simulink model "Semi_Lead_Guidance_Method_6"  (R2024b)
settings: Solver=FixedStepAuto  StartTime=0.0  StopTime=200  FixedStep=0.01  RelTol=1e-3
values from neighbouring files (symbols this model uses):
  P = 2    [AAZ.m]    (also in TP3_1_6.m = P_values(idx))
settings Model: Creator=Acer  LastModifiedBy=Acer
settings DataIOCC: ReturnWorkspaceOutputs=off

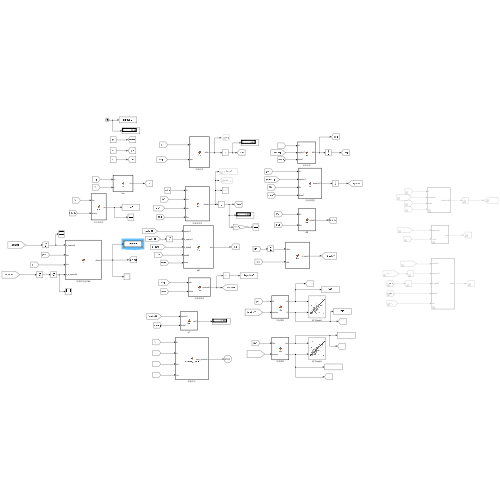
[thumbnail: Simulink's stored preview of the top-level diagram]
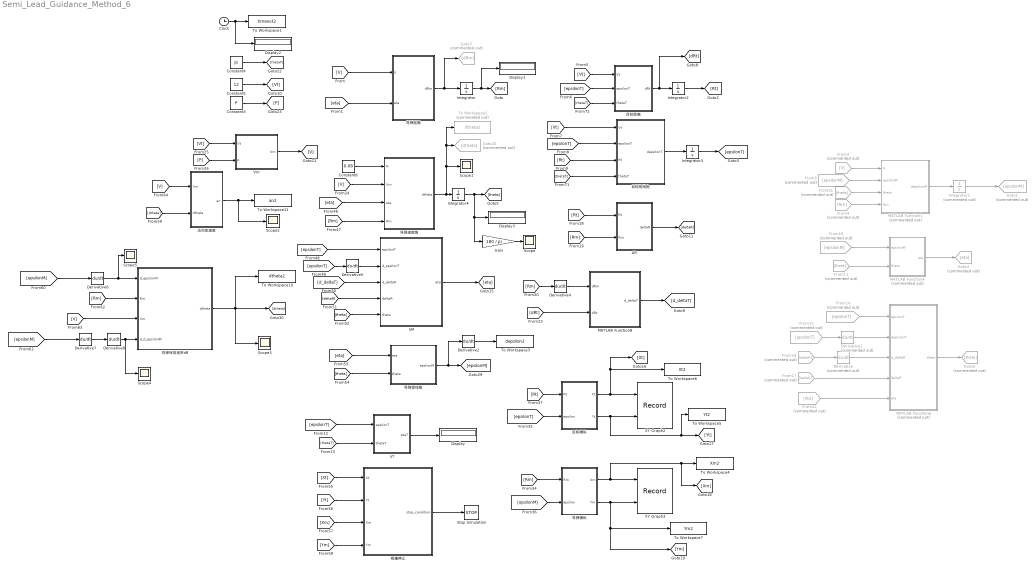
== system Semi_Lead_Guidance_Method_6 ==
  Clock : Clock
  Constant3 : Constant  Value=P
  Constant4 : Constant  Value=pi
  Constant5 : Constant  Value=12
  Constant6 : Constant  Value=0.08
  Derivative : Derivative  Commented=on
  Derivative1 : Derivative  Commented=on
  Derivative{2,4..8} (6 alike) : Derivative
  Display{,1..3} (4 alike) : Display
  From10 : From  Commented=on  GotoTag=epsilonM
  From11 : From  Commented=on  GotoTag=theta
  From14 : From  Commented=on  GotoTag=epsilonT
  From15 : From  Commented=on  GotoTag=epsilonT
  From16 : From  Commented=on  GotoTag=deltaR
  From17 : From  Commented=on  GotoTag=deltaR
  From2 : From  Commented=on  GotoTag=V
  From21 : From  Commented=on  GotoTag=theta
  From22 : From  Commented=on  GotoTag=eta
  From3 : From  Commented=on  GotoTag=epsilonM
  From4 : From  Commented=on  GotoTag=Rm
  Gain : Gain  Gain=180 / pi
  Goto1 : Goto  Commented=on  GotoTag=epsilonM
  Goto20 : Goto  Commented=on  GotoTag=dtheta
  Goto4 : Goto  Commented=on  GotoTag=eta
  Goto6 : Goto  Commented=on  GotoTag=theta
  Goto7 : Goto  Commented=on  GotoTag=dRm
  Integrator : Integrator  InitialCondition=50
  Integrator1 : Integrator  Commented=on  InitialCondition=65*pi/180
  Integrator2 : Integrator  InitialCondition=3000
  Integrator3 : Integrator  InitialCondition=70 * pi / 180
  Integrator4 : Integrator  InitialCondition=70 * pi /180
  MATLAB Function1 : MATLAB Function  Commented=on  TreatAsAtomicUnit=on
  MATLAB Function4 : MATLAB Function  Commented=on  TreatAsAtomicUnit=on
  MATLAB Function6 : MATLAB Function  Commented=on  TreatAsAtomicUnit=on
  MATLAB Function8 : MATLAB Function  TreatAsAtomicUnit=on
  Scope{,1..5} (6 alike) : Scope
  Stop Simulation : Stop
  To Workspace1 : ToWorkspace  VariableName=timeout2  SaveFormat=Timeseries  SampleTime=-1
  To Workspace10 : ToWorkspace  VariableName=dtheta2  SaveFormat=Timeseries  SampleTime=-1
  To Workspace11 : ToWorkspace  VariableName=an2  SaveFormat=Timeseries  SampleTime=-1
  To Workspace2 : ToWorkspace  Commented=on  VariableName=dtheta2  SaveFormat=Timeseries  SampleTime=-1
  To Workspace3 : ToWorkspace  VariableName=depsilon2  SaveFormat=Timeseries  SampleTime=-1
  To Workspace4 : ToWorkspace  VariableName=Xm2  SaveFormat=Timeseries  SampleTime=-1
  To Workspace5 : ToWorkspace  VariableName=Yt2  SaveFormat=Timeseries  SampleTime=-1
  To Workspace6 : ToWorkspace  VariableName=Xt2  SaveFormat=Timeseries  SampleTime=-1
  To Workspace7 : ToWorkspace  VariableName=Ym2  SaveFormat=Timeseries  SampleTime=-1
  Vm : MATLAB Function  TreatAsAtomicUnit=on
  XY Graph2 : Record  FileSettingsInternal="{\"entries\":[{\"content\":{\"excelSettings\":{\"content\":{},\"type\":\"Streamout.ExcelSettings\"}},\"type\":\"Streamout.FileSettingStorage\",\"uuid\":\"\"}],\"packageUris\":[\"http:\\/\\/schema.mathworks.com\\/mf0\\/streamout_blocks\\/R2020a\"],\"version\":\"1.0\"}"  Layout=[1 1]  SignalsInternal="{\"entries\":[{\"content\":{\"signals\":[{\"content\":{\"blockPath\":[],\"dimensions\":[1],\"domain\":\"\",\"lineColor\":\"#b746ff\",\"lineWidth\":2,\"plots\":[ 1 ],\"port\":1,\"sid\":[\"\"],\"signalID\":1,\"signalName\":\"目标横纵:1\"},\"type\":\"RecordBlkView.Signal\",\"uuid\":\"\"},{\"content\":{\"blockPath\":[],\"dimensions\":[1],\"domain\":\"\",\"lineColor\":\"#64d413\",\"lineWidth\":2,\"plots\":[ 1 ],\"port\":2,\"sid\":[\"\"],\"signalID\":2,\"signalName\":\"目标横纵:2\"},\"type\":\"RecordBlkView.Signal\",\"uuid\":\"\"}]},\"type\":\"RecordBlkView.InputSignals\",\"uuid\":\"\"}],\"packageUris\":[\"http:\\/\\/schema.mathworks.com\\/mf0\\/streamout_blocks\\/R2020a\"],\"version\":\"1.0\"}"  VisualizationBindings="{\"xyplotplugin\":{\"info\":[{\"series\":[{\"bindingParametersList\":[{\"parameter\":\"X-Axis\",\"signalID\":1,\"signalName\":\"目标横纵:1\"},{\"parameter\":\"Y-Axis\",\"signalID\":2,\"signalName\":\"目标横纵:2\"}],\"seriesID\":0}],\"subplotID\":1}]}}"  CompatibilityTag=XY
  XY Graph3 : Record  FileSettingsInternal="{\"entries\":[{\"content\":{\"excelSettings\":{\"content\":{},\"type\":\"Streamout.ExcelSettings\"}},\"type\":\"Streamout.FileSettingStorage\",\"uuid\":\"\"}],\"packageUris\":[\"http:\\/\\/schema.mathworks.com\\/mf0\\/streamout_blocks\\/R2020a\"],\"version\":\"1.0\"}"  Layout=[1 1]  SignalsInternal="{\"entries\":[{\"content\":{\"signals\":[{\"content\":{\"blockPath\":[],\"dimensions\":[1],\"domain\":\"\",\"lineColor\":\"#ff13a6\",\"lineWidth\":2,\"plots\":[ 1 ],\"port\":1,\"sid\":[\"\"],\"signalID\":1,\"signalName\":\"导弹横纵:1\"},\"type\":\"RecordBlkView.Signal\",\"uuid\":\"\"},{\"content\":{\"blockPath\":[],\"dimensions\":[1],\"domain\":\"\",\"lineColor\":\"#fe330a\",\"lineWidth\":2,\"plots\":[ 1 ],\"port\":2,\"sid\":[\"\"],\"signalID\":2,\"signalName\":\"导弹横纵:2\"},\"type\":\"RecordBlkView.Signal\",\"uuid\":\"\"}]},\"type\":\"RecordBlkView.InputSignals\",\"uuid\":\"\"}],\"packageUris\":[\"http:\\/\\/schema.mathworks.com\\/mf0\\/streamout_blocks\\/R2020a\"],\"version\":\"1.0\"}"  VisualizationBindings="{\"xyplotplugin\":{\"info\":[{\"series\":[{\"bindingParametersList\":[{\"parameter\":\"X-Axis\",\"signalID\":1,\"signalName\":\"导弹横纵:1\"},{\"parameter\":\"Y-Axis\",\"signalID\":2,\"signalName\":\"导弹横纵:2\"}],\"seriesID\":0}],\"subplotID\":1}]}}"  CompatibilityTag=XY
  ΔR : MATLAB Function  TreatAsAtomicUnit=on
  ηM : MATLAB Function  TreatAsAtomicUnit=on
  ηT : MATLAB Function  TreatAsAtomicUnit=on
  导弹横纵 : MATLAB Function  TreatAsAtomicUnit=on
  导弹视线角 : MATLAB Function  TreatAsAtomicUnit=on
  导弹距离 : MATLAB Function  TreatAsAtomicUnit=on
  导弹转弯速率dθ : MATLAB Function  TreatAsAtomicUnit=on
  导弹速度角 : MATLAB Function  TreatAsAtomicUnit=on
  法向加速度 : MATLAB Function  TreatAsAtomicUnit=on
  目标横纵 : MATLAB Function  TreatAsAtomicUnit=on
  目标视线角 : MATLAB Function  TreatAsAtomicUnit=on
  目标距离 : MATLAB Function  TreatAsAtomicUnit=on
  相撞停止 : MATLAB Function  TreatAsAtomicUnit=on
  wires:
  [Rm] -> ΔR/2(Rm)
  [Ym] -> 相撞停止/4(Ym)
  [epsilonT] -> Derivative5/1
  Derivative1/1 -> MATLAB Function6/2(depsilonT)
  Derivative/1 -> MATLAB Function6/3(d_deltaR)
  [eta] -> 导弹距离/2(eta)
  [Xt] -> 相撞停止/1(Xt)
  ηT/1(etaT) -> Display/1
  [eta] -> 导弹视线角/1(eta)
  [Rt] -> 目标横纵/1(Rt)
  导弹视线角/1(epsilonM) -> Derivative2/1, [epsilonM]
  目标横纵/1(Xt) -> XY Graph2/1, To Workspace6/1, [Xt]
  Derivative5/1 -> ηM/2(d_epsilonT)
  Integrator4/1 -> Gain/1, Display3/1, [theta]
  目标横纵/2(Yt) -> To Workspace5/1, [Yt], XY Graph2/2
  导弹距离/1(dRm) -> Goto7/1, Integrator/1
  [V] -> 导弹距离/1(V)
  From2/1 -> MATLAB Function1/1(V)
  [eta] -> 导弹速度角/3(eta)
  From17/1 -> MATLAB Function6/4(deltaR)
  [Xm] -> 相撞停止/3(Xm)
  导弹横纵/2(Ym) -> [Ym], To Workspace7/1, XY Graph3/2
  [epsilonT] -> ηT/1(epsilonT)
  MATLAB Function8/1(d_deltaT) -> [d_deltaT]
  From14/1 -> MATLAB Function6/1(epsilonT)
  [thetaT] -> ηT/2(thetaT)
  Integrator/1 -> Display1/1, [Rm]
  [theta] -> ηM/5(theta)
  [Rm] -> Derivative4/1
  ΔR/1(deltaR) -> [deltaR]
  From3/1 -> MATLAB Function1/2(epsilonM)
  [deltaR] -> ηM/4(deltaR)
  MATLAB Function1/1(depsilonM) -> Integrator1/1
  [epsilonM] -> 导弹横纵/2(epsilon)
  From15/1 -> Derivative1/1
  From10/1 -> MATLAB Function4/1(epsilonM)
  [theta] -> 导弹视线角/2(theta)
  [epsilonT] -> ηM/1(epsilonT)
  Constant6/1 -> 导弹速度角/1(N)
  MATLAB Function6/1(theta) -> Goto6/1
  Clock/1 -> Display2/1, To Workspace1/1
  [dRt] -> MATLAB Function8/2(dRt)
  MATLAB Function4/1(eta) -> Goto4/1
  导弹速度角/1(dtheta) -> To Workspace2/1, Goto20/1, Scope1/1, Integrator4/1
  [Rt] -> ΔR/1(Rt)
  导弹横纵/1(Xm) -> [Xm], To Workspace4/1, XY Graph3/1
  [Rm] -> 导弹速度角/4(Rm)
  From22/1 -> MATLAB Function6/5(eta)
  [d_deltaT] -> ηM/3(d_deltaR)
  From11/1 -> MATLAB Function4/2(theta)
  Integrator1/1 -> Goto1/1
  [Rm] -> 导弹横纵/1(Rm)
  Derivative4/1 -> MATLAB Function8/1(dRm)
  相撞停止/1(stop_condition) -> Stop Simulation/1
  [Yt] -> 相撞停止/2(Yt)
  From16/1 -> Derivative/1
  From21/1 -> MATLAB Function1/3(theta)
  From4/1 -> MATLAB Function1/4(Rm)
  [V] -> 导弹速度角/2(Vm)
  ηM/1(eta) -> [eta]
  [epsilonT] -> 目标横纵/2(epsilon)
  [V] -> 法向加速度/1(Vm)
  [dtheta] -> 法向加速度/2(dtheta)
  法向加速度/1(an) -> Scope2/1, To Workspace11/1
  Gain/1 -> Scope/1
  Derivative2/1 -> To Workspace3/1
  [thetaT] -> 目标距离/3(thetaT)
  [Rt] -> 目标视线角/3(Rt)
  目标视线角/1(depsilonT) -> Integrator3/1
  [Vt] -> 目标视线角/1(Vt)
  目标距离/1(dRt) -> Integrator2/1, [dRt]
  [epsilonT] -> 目标视线角/2(epsilonT)
  Integrator2/1 -> [Rt]
  Integrator3/1 -> [epsilonT]
  [Vt] -> 目标距离/1(Vt)
  [epsilonT] -> 目标距离/2(epsilonT)
  [thetaT] -> 目标视线角/4(thetaT)
  [Vt] -> Vm/1(Vt)
  Constant3/1 -> [P]
  [P] -> Vm/2(p)
  Constant5/1 -> [Vt]
  Constant4/1 -> [thetaT]
  Vm/1(Vm) -> [V]
  Derivative6/1 -> Scope5/1, 导弹转弯速率dθ/1(d_epsilonM)
  Derivative8/1 -> Scope4/1, 导弹转弯速率dθ/4(d_d_epsilonM)
  [epsilonM] -> Derivative6/1
  Derivative7/1 -> Derivative8/1
  [Rm] -> 导弹转弯速率dθ/2(Rm)
  导弹转弯速率dθ/1(dtheta) -> To Workspace10/1, Scope3/1, [dtheta]
  [epsilonM] -> Derivative7/1
  [V] -> 导弹转弯速率dθ/3(Vm)

== matlab function Semi_Lead_Guidance_Method_6/Vm ==
  data: Vt input; Vm output; p input
function Vm = fcn(Vt, p)

Vm = Vt * p;

== matlab function Semi_Lead_Guidance_Method_6/目标横纵 ==
  data: Rt input; Xt output; epsilon input; Yt output
function [Xt, Yt] = fcn(Rt, epsilon)

Xt = Rt * cos(epsilon);
Yt = Rt * sin(epsilon);

== matlab function Semi_Lead_Guidance_Method_6/导弹横纵 ==
  data: Rm input; Xm output; epsilon input; Ym output
function [Xm, Ym] = fcn(Rm, epsilon)

Xm = Rm * cos(epsilon);
Ym = Rm * sin(epsilon);

== matlab function Semi_Lead_Guidance_Method_6/ηM ==
  data: eta output; epsilonT input; d_epsilonT input; d_deltaR input; deltaR input; theta input
function eta = fcn(epsilonT, d_epsilonT, d_deltaR, deltaR, theta)

    eta = epsilonT - 0.5 * (d_epsilonT * deltaR / d_deltaR) - theta;
end

== matlab function Semi_Lead_Guidance_Method_6/导弹视线角 ==
  data: eta input; epsilonM output; theta input
function epsilonM = fcn(eta, theta)

epsilonM = eta + theta;

== matlab function Semi_Lead_Guidance_Method_6/相撞停止 ==
  data: Xt input; stop_condition output; Yt input; Xm input; Ym input
function stop_condition = distance_check(Xt, Yt, Xm, Ym)
    
    distance = sqrt((Xt - Xm)^2 + (Yt - Ym)^2);
    stop_condition = distance < 1;
    
end

== matlab function Semi_Lead_Guidance_Method_6/MATLAB Function1 ==
  data: V input; depsilonM output; epsilonM input; theta input; Rm input
function depsilonM = fcn(V, epsilonM, theta, Rm)

    depsilonM = -(V * sin(epsilonM - theta) / Rm);
end

== matlab function Semi_Lead_Guidance_Method_6/导弹转弯速率dθ ==
  data: d_epsilonM input; Rm input; Vm input; d_d_epsilonM input; dtheta output
function dtheta = fcn(d_epsilonM, Rm, Vm, d_d_epsilonM)
    dtheta = 2 * d_epsilonM + Rm * d_d_epsilonM/ Vm;
end

== matlab function Semi_Lead_Guidance_Method_6/法向加速度 ==
  data: Vm input; an output; dtheta input
function an = fcn(Vm, dtheta)
    an = Vm * dtheta;
end

== matlab function Semi_Lead_Guidance_Method_6/导弹距离 ==
  data: V input; dRm output; eta input
function dRm = fcn(V, eta)

    dRm = V * cos(eta);
end

== matlab function Semi_Lead_Guidance_Method_6/目标距离 ==
  data: Vt input; dRt output; epsilonT input; thetaT input
function dRt = fcn(Vt, epsilonT, thetaT)

    dRt = Vt * cos(epsilonT - thetaT);
end

== matlab function Semi_Lead_Guidance_Method_6/目标视线角 ==
  data: Vt input; depsilonT output; epsilonT input; Rt input; thetaT input
function depsilonT = fcn(Vt, epsilonT, Rt, thetaT)

    depsilonT = - ((Vt * sin(epsilonT - thetaT)) / Rt);
end

== matlab function Semi_Lead_Guidance_Method_6/MATLAB Function4 ==
  data: epsilonM input; eta output; theta input
function eta = fcn(epsilonM, theta)

eta = epsilonM - theta;

== matlab function Semi_Lead_Guidance_Method_6/ηT ==
  data: epsilonT input; etaT output; thetaT input
function etaT = fcn(epsilonT, thetaT)

etaT = epsilonT - thetaT;

== matlab function Semi_Lead_Guidance_Method_6/MATLAB Function6 ==
  data: epsilonT input; theta output; depsilonT input; d_deltaR input; deltaR input; eta input
function theta = fcn(epsilonT, depsilonT, d_deltaR, deltaR, eta)

theta = epsilonT - ((depsilonT / d_deltaR ) * deltaR) - eta;

== matlab function Semi_Lead_Guidance_Method_6/ΔR ==
  data: Rt input; deltaR output; Rm input
function deltaR = fcn(Rt, Rm)

deltaR = Rt - Rm;

== matlab function Semi_Lead_Guidance_Method_6/MATLAB Function8 ==
  data: dRm input; d_deltaT output; dRt input
function d_deltaT = fcn(dRm, dRt)

d_deltaT = dRt - dRm;

== matlab function Semi_Lead_Guidance_Method_6/导弹速度角 ==
  data: N input; dtheta output; Vm input; eta input; Rm input
function dtheta = fcn(N, Vm, eta, Rm)

dtheta = (-N) * Vm * sin(eta) / Rm;
